simulink model "all_link_models"  (R2018a)
settings: Solver=VariableStepDiscrete  StartTime=0.0  StopTime=250  RelTol=1e-3  EnableMultiTasking=on
libraries: commchan3 x4, commdigbbndpm3 x4, commrandsrc3 x4, commsink2 x4, commdigbbndfm2 x2, commdigbbndam3 x2
settings Model: ExtModeAutoUpdateStatusClock=off  Creator=The MathWorks, Inc.  LastModifiedBy=erictanner
settings DataIOCC: LimitDataPoints=on  SaveFormat=Array  SignalLoggingName=sigsOut
settings OptimizationCC: BlockReduction=off  BooleanDataType=off  ExpressionDepthLimit=2147483647  InitFltsAndDblsToZero=on  LifeSpan=inf
settings DebuggingCC: SaveWithParameterizedLinksMsg=none  UnderspecifiedInitializationDetection=Classic  MergeDetectMultiDrivingBlocksExec=none  CheckExecutionContextPreStartOutputMsg=on  CheckExecutionContextRuntimeOutputMsg=on  SignalResolutionControl=TryResolveAllWithWarning  InheritedTsInSrcMsg=none  MultiTaskDSMMsg=warning  MultiTaskCondExecSysMsg=none  FcnCallInpInsideContextMsg=warning  StateNameClashWarn=warning  SFUnexpectedBacktrackingDiag=warning  SFNoUnconditionalDefaultTransitionDiag=warning  SFExecutionAtInitializationDiag=none
settings HardwareCC: ProdBitPerPointer=32  ProdBitPerSizeT=32  ProdBitPerPtrDiffT=32  ProdLargestAtomicFloat=None  ProdIntDivRoundTo=Undefined  ProdEndianess=Unspecified  ProdWordSize=32  ProdHWDeviceType=32-bit Generic  TargetUnknown=on
settings ModelReferenceCC: UpdateModelReferenceTargets=IfOutOfDate  PropagateSignalLabelsOutOfModel=off
settings CodeAppCC: StateflowObjectComments=on
settings GRTTargetCC: TargetFcnLib=ansi_tfl_tmw.mat  TargetLangStandard=C89/C90 (ANSI)  GeneratePreprocessorConditionals=Disable all  CombineOutputUpdateFcns=off  GRTInterface=on
settings ConfigComp: CovMetricSettings=dw  CovHtmlReporting=on  CovSaveCumulativeToWorkspaceVar=on  CovSaveSingleToWorkspaceVar=on  CovExternalEMLEnable=off

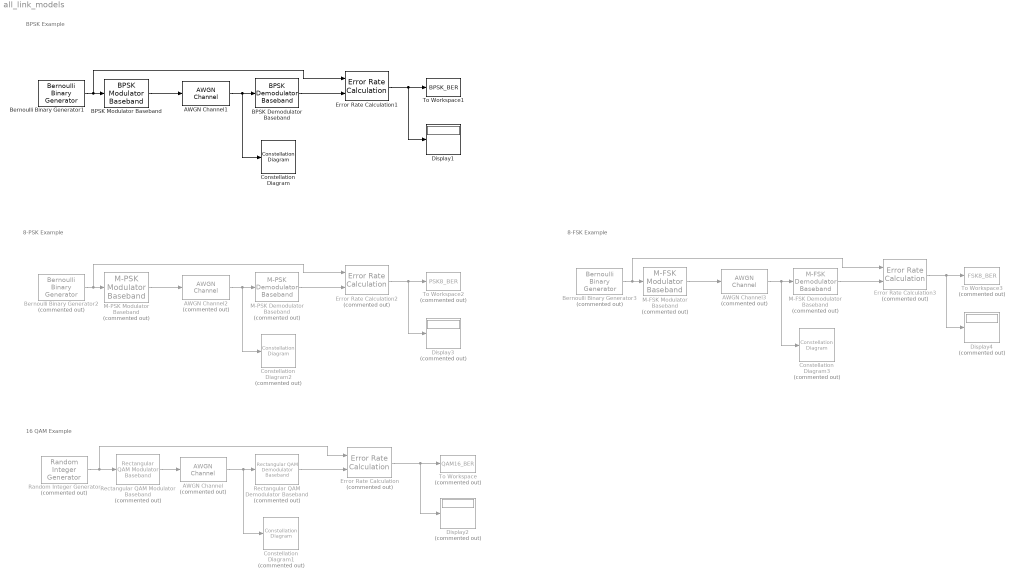
== system all_link_models ==
  note: 16 QAM Example
  note: BPSK Example
  note: 8-PSK Example
  note: 8-FSK Example
  AWGN Channel : commchan3/AWGN Channel  Commented=on  InputProcessing=Columns as channels (frame based)  seed=1  noiseMode="Signal to noise ratio  (SNR)"  EbNodB=10  EsNodB=50  SNRdB=20  bitsPerSym=1  Ps=1  Tsym=.1  variance=1
  AWGN Channel1 : commchan3/AWGN Channel  InputProcessing=Columns as channels (frame based)  seed=37  noiseMode="Signal to noise ratio  (SNR)"  EbNodB=40  EsNodB=20  SNRdB=8  bitsPerSym=1  Ps=1  Tsym=100  variance=1
  AWGN Channel2 : commchan3/AWGN Channel  Commented=on  InputProcessing=Columns as channels (frame based)  seed=1  noiseMode="Signal to noise ratio  (SNR)"  EbNodB=10  EsNodB=20  SNRdB=20  bitsPerSym=1  Ps=1  Tsym=.1  variance=1
  AWGN Channel3 : commchan3/AWGN Channel  Commented=on  InputProcessing=Columns as channels (frame based)  seed=1  noiseMode="Signal to noise ratio  (SNR)"  EbNodB=10  EsNodB=20  SNRdB=20  bitsPerSym=1  Ps=1  Tsym=.1  variance=1
  BPSK Demodulator Baseband : commdigbbndpm3/BPSK Demodulator Baseband  DecType=Hard decision  VarSource=Dialog  Variance=1  Ph=0  outDtype=Inherit via internal rule  derotateFactorWordLen=16  derotateFactorDataTypeStr=Inherit: Same word length as input  derotateFactorLastDataTypeStr=Inherit: Same word length as input
  BPSK Modulator Baseband : commdigbbndpm3/BPSK Modulator Baseband  Ph=0  outDtype=Inherit via back propagation  outWordLen=16  outUDDataType=sfix(16)  outFracLenMode=Best precision  outFracLen=15  outDataTypeStr=Inherit: Inherit via back propagation  outLastDataTypeStr=Inherit: Inherit via back propagation
  Bernoulli Binary Generator1 : commrandsrc3/Bernoulli Binary Generator  ProbabilityOfZero=0.5  SeedSource=Parameter  Seed=61  SampleTime=0.01  SamplesPerFrame=1  OutputDataType=double  SimulateUsing=Interpreted execution
  Bernoulli Binary Generator2 : commrandsrc3/Bernoulli Binary Generator  Commented=on  ProbabilityOfZero=0.5  SeedSource=Parameter  Seed=61  SampleTime=1  SamplesPerFrame=1000  OutputDataType=double  SimulateUsing=Interpreted execution
  Bernoulli Binary Generator3 : commrandsrc3/Bernoulli Binary Generator  Commented=on  ProbabilityOfZero=0.5  SeedSource=Parameter  Seed=61  SampleTime=1  SamplesPerFrame=1000  OutputDataType=double  SimulateUsing=Interpreted execution
  Constellation Diagram : ConstellationDiagram
  Constellation Diagram1 : ConstellationDiagram  Commented=on
  Constellation Diagram2 : ConstellationDiagram  Commented=on
  Constellation Diagram3 : ConstellationDiagram  Commented=on
  Display1 : Display
  Display2 : Display  Commented=on
  Display3 : Display  Commented=on
  Display4 : Display  Commented=on
  Error Rate Calculation : commsink2/Error Rate Calculation  Commented=on  N=0  st_delay=0  cp_mode=Entire frame  subframe=[]  PMode=Port  WsName=QAM16_ErrorVec  RsMode2=off  stop=off  numErr=100  maxBits=1e6
  Error Rate Calculation1 : commsink2/Error Rate Calculation  N=0  st_delay=0  cp_mode=Entire frame  subframe=[]  PMode=Port  WsName=BPSK_ErrorVec  RsMode2=off  stop=on  numErr=100  maxBits=1e4
  Error Rate Calculation2 : commsink2/Error Rate Calculation  Commented=on  N=0  st_delay=0  cp_mode=Entire frame  subframe=[]  PMode=Port  WsName=BPSK_ErrorVec  RsMode2=off  stop=off  numErr=100  maxBits=1e6
  Error Rate Calculation3 : commsink2/Error Rate Calculation  Commented=on  N=0  st_delay=0  cp_mode=Entire frame  subframe=[]  PMode=Port  WsName=BPSK_ErrorVec  RsMode2=off  stop=off  numErr=100  maxBits=1e6
  M-FSK Demodulator Baseband : commdigbbndfm2/M-FSK Demodulator Baseband  Commented=on  M=8  OutType=Integer  Dec=Gray  freqSep=6  numSamp=17  RateOptions=Enforce single-rate processing  outDataType=double
      settings: SourceProductName=Communications System Toolbox  SourceProductBaseCode=CM
  M-FSK Modulator Baseband : commdigbbndfm2/M-FSK Modulator Baseband  Commented=on  M=8  InType=Integer  Enc=Gray  freqSep=6  phaseType=Continuous  numSamp=17  RateOptions=Enforce single-rate processing  outDataType=double
      settings: SourceProductName=Communications System Toolbox
  M-PSK Demodulator Baseband : commdigbbndpm3/M-PSK Demodulator Baseband  Commented=on  M=8  OutType=Integer  DecType=Hard decision  VarSource=Dialog  Variance=1  Dec=Gray  Mapping=[0:7]  Ph=pi/8  outDtype1=Inherit via internal rule  outDtype2=Inherit via internal rule  derotateFactorWordLen=16  derotateFactorDataTypeStr=Inherit: Same word length as input  derotateFactorLastDataTypeStr=Inherit: Same word length as input
      settings: SourceProductName=Communications System Toolbox
  M-PSK Modulator Baseband : commdigbbndpm3/M-PSK Modulator Baseband  Commented=on  M=8  InType=Integer  Enc=Gray  Mapping=[0:7]  Ph=pi/8  outDtype=double  outWordLen=16  outUDDataType=sfix(16)  outFracLenMode=Best precision  outFracLen=15  outDataTypeStr=double  outLastDataTypeStr=double
      settings: SourceProductName=Communications System Toolbox
  Random Integer Generator : commrandsrc3/Random Integer Generator  Commented=on  SetSize=16  SeedSource=Auto  Seed=392  SampleTime=1  SamplesPerFrame=1000  OutputDataType=double  SimulateUsing=Interpreted execution
  Rectangular QAM Demodulator Baseband : commdigbbndam3/Rectangular QAM Demodulator Baseband  Commented=on  M=16  OutType=Integer  DecType=Hard decision  VarSource=Dialog  Variance=1  Dec=Binary  Mapping=[0:15]  PowType=Peak Power  MinDist=2  AvgPow=1  PeakPow=1  Ph=0  outDtype1=Inherit via internal rule  outDtype2=Inherit via internal rule  derotateFactorWordLen=16  derotateFactorDataTypeStr=Inherit: Same word length as input  derotateFactorLastDataTypeStr=Inherit: Same word length as input  denormFactorWordLen=16  denormFactorDataTypeStr=Inherit: Same word length as input  denormFactorLastDataTypeStr=Inherit: Same word length as input  prodOutWordLen=32  prodOutOverflowMode=Wrap  prodOutRoundingMode=Floor  prodOutOvFlMode=off  prodOutOvFlModeLastStrValue=off  sumWordLen=32
  Rectangular QAM Modulator Baseband : commdigbbndam3/Rectangular QAM Modulator Baseband  Commented=on  M=16  InType=Integer  Enc=Binary  Mapping=[0:15]  PowType=Peak Power  MinDist=2  AvgPow=1  PeakPow=1  Ph=0  outDtype=double  outWordLen=16  outUDDataType=sfix(16)  outFracLenMode=Best precision  outFracLen=15  outDataTypeStr=double  outLastDataTypeStr=double
  To Workspace : ToWorkspace  Commented=on  VariableName=QAM16_BER  SampleTime=-1
      settings: MaxDataPoints=1  Save2DSignal=2-D array (concatenate along first dimension)
  To Workspace1 : ToWorkspace  VariableName=BPSK_BER  SampleTime=-1
      settings: MaxDataPoints=1  Save2DSignal=2-D array (concatenate along first dimension)
  To Workspace2 : ToWorkspace  Commented=on  VariableName=PSK8_BER  SampleTime=-1
      settings: MaxDataPoints=1  Save2DSignal=2-D array (concatenate along first dimension)
  To Workspace3 : ToWorkspace  Commented=on  VariableName=FSK8_BER  SampleTime=-1
      settings: MaxDataPoints=1  Save2DSignal=2-D array (concatenate along first dimension)
  wires:
  Random Integer Generator/1 -> Error Rate Calculation/1, Rectangular QAM Modulator Baseband/1
  BPSK Modulator Baseband/1 -> AWGN Channel1/1
  Bernoulli Binary Generator1/1 -> Error Rate Calculation1/1, BPSK Modulator Baseband/1
  Rectangular QAM Demodulator Baseband/1 -> Error Rate Calculation/2
  BPSK Demodulator Baseband/1 -> Error Rate Calculation1/2
  Error Rate Calculation/1 -> Display2/1, To Workspace/1
  Error Rate Calculation1/1 -> Display1/1, To Workspace1/1
  Rectangular QAM Modulator Baseband/1 -> AWGN Channel/1
  AWGN Channel1/1 -> BPSK Demodulator Baseband/1, Constellation Diagram/1
  AWGN Channel/1 -> Rectangular QAM Demodulator Baseband/1, Constellation Diagram1/1
  Bernoulli Binary Generator2/1 -> M-PSK Modulator Baseband/1, Error Rate Calculation2/1
  M-PSK Modulator Baseband/1 -> AWGN Channel2/1
  Error Rate Calculation2/1 -> Display3/1, To Workspace2/1
  AWGN Channel2/1 -> M-PSK Demodulator Baseband/1, Constellation Diagram2/1
  M-PSK Demodulator Baseband/1 -> Error Rate Calculation2/2
  Bernoulli Binary Generator3/1 -> M-FSK Modulator Baseband/1, Error Rate Calculation3/1
  M-FSK Modulator Baseband/1 -> AWGN Channel3/1
  Error Rate Calculation3/1 -> Display4/1, To Workspace3/1
  AWGN Channel3/1 -> M-FSK Demodulator Baseband/1, Constellation Diagram3/1
  M-FSK Demodulator Baseband/1 -> Error Rate Calculation3/2
